simulink model "Conduction_Losses"  (R2015a)
settings: Solver=ode45  StartTime=0.0  StopTime=10.0  RelTol=1e-3
libraries: simulink x6
settings Model: Creator=Caner  LastModifiedBy=Caner

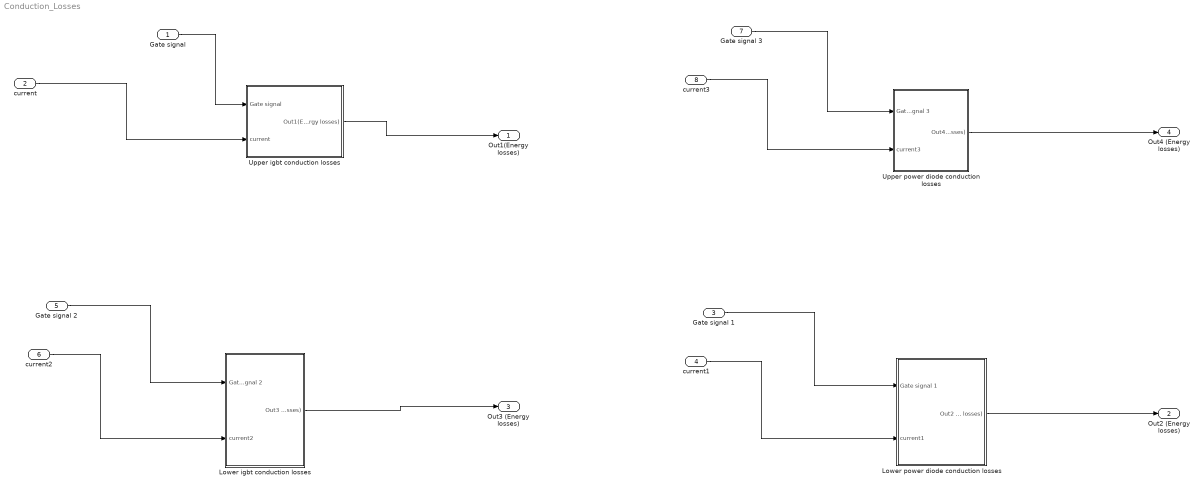
== system Conduction_Losses ==
  "Gate signal " : Inport
  current : Inport  Port=2
  Gate signal 1 : Inport  Port=3
  current1 : Inport  Port=4
  Gate signal 2 : Inport  Port=5
  current2 : Inport  Port=6
  Gate signal 3 : Inport  Port=7
  current3 : Inport  Port=8
  Lower igbt conduction losses : Subsystem
  Lower power diode conduction losses : Subsystem
  Upper igbt conduction losses : Subsystem
  Upper power diode conduction losses : Subsystem
  Out1(Energy losses) : Outport
  Out2 (Energy losses) : Outport  Port=2
  Out3 (Energy losses) : Outport  Port=3
  Out4 (Energy losses) : Outport  Port=4
  wires:
  "Gate signal "/1 -> Upper igbt conduction losses/1("Gate signal ")
  current/1 -> Upper igbt conduction losses/2(current)
  Upper igbt conduction losses/1(Out1(Energy losses)) -> Out1(Energy losses)/1
  Gate signal 2/1 -> Lower igbt conduction losses/1(Gate signal 2)
  current2/1 -> Lower igbt conduction losses/2(current2)
  Lower igbt conduction losses/1(Out3 (Energy losses)) -> Out3 (Energy losses)/1
  Gate signal 3/1 -> Upper power diode conduction losses/1(Gate signal 3)
  current3/1 -> Upper power diode conduction losses/2(current3)
  Upper power diode conduction losses/1(Out4 (Energy losses)) -> Out4 (Energy losses)/1
  Gate signal 1/1 -> Lower power diode conduction losses/1(Gate signal 1)
  current1/1 -> Lower power diode conduction losses/2(current1)
  Lower power diode conduction losses/1(Out2 (Energy losses)) -> Out2 (Energy losses)/1

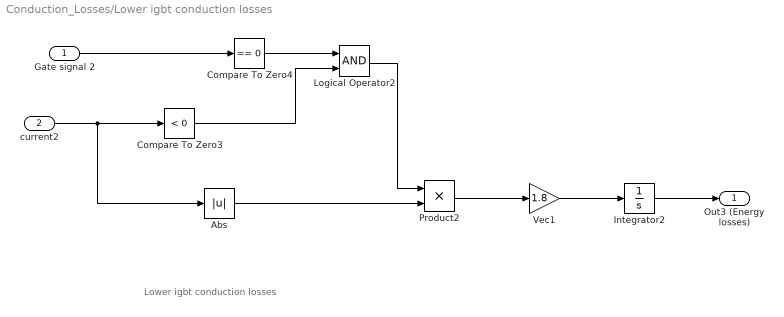
== system Conduction_Losses/Lower igbt conduction losses ==
  note: Lower igbt conduction losses
  Gate signal 2 : Inport
  current2 : Inport  Port=2
  Abs : Abs
  Compare To Zero3 : simulink/Logic and Bit Operations/Compare To Zero  relop=<  OutDataTypeStr=boolean
  Compare To Zero4 : simulink/Logic and Bit Operations/Compare To Zero  relop===  OutDataTypeStr=boolean
  Integrator2 : Integrator
  Logical Operator2 : Logic  AllPortsSameDT=off  OutDataTypeStr=boolean
  Product2 : Product
  Vec1 : Gain  Gain=1.8
  Out3 (Energy losses) : Outport
  wires:
  Gate signal 2/1 -> Compare To Zero4/1
  Compare To Zero3/1 -> Logical Operator2/2
  current2/1 -> Abs/1, Compare To Zero3/1
  Vec1/1 -> Integrator2/1
  Abs/1 -> Product2/2
  Compare To Zero4/1 -> Logical Operator2/1
  Product2/1 -> Vec1/1
  Integrator2/1 -> Out3 (Energy losses)/1
  Logical Operator2/1 -> Product2/1

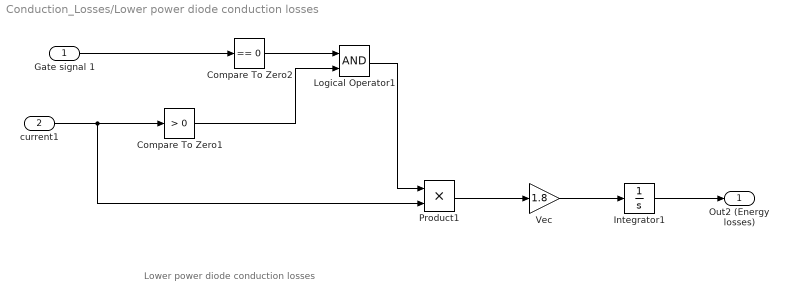
== system Conduction_Losses/Lower power diode conduction losses ==
  note: Lower power diode conduction losses
  Gate signal 1 : Inport
  current1 : Inport  Port=2
  Compare To Zero1 : simulink/Logic and Bit Operations/Compare To Zero  relop=>  OutDataTypeStr=boolean
  Compare To Zero2 : simulink/Logic and Bit Operations/Compare To Zero  relop===  OutDataTypeStr=boolean
  Integrator1 : Integrator
  Logical Operator1 : Logic  AllPortsSameDT=off  OutDataTypeStr=boolean
  Product1 : Product
  Vec : Gain  Gain=1.8
  Out2 (Energy losses) : Outport
  wires:
  Compare To Zero1/1 -> Logical Operator1/2
  Logical Operator1/1 -> Product1/1
  Gate signal 1/1 -> Compare To Zero2/1
  current1/1 -> Product1/2, Compare To Zero1/1
  Compare To Zero2/1 -> Logical Operator1/1
  Vec/1 -> Integrator1/1
  Integrator1/1 -> Out2 (Energy losses)/1
  Product1/1 -> Vec/1

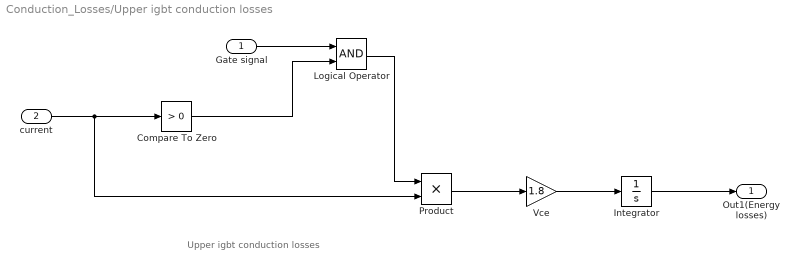
== system Conduction_Losses/Upper igbt conduction losses ==
  note: Upper igbt conduction losses
  "Gate signal " : Inport
  current : Inport  Port=2
  Compare To Zero : simulink/Logic and Bit Operations/Compare To Zero  relop=>  OutDataTypeStr=boolean
  Integrator : Integrator
  Logical Operator : Logic  AllPortsSameDT=off  OutDataTypeStr=boolean
  Product : Product
  Vce : Gain  Gain=1.8
  Out1(Energy losses) : Outport
  wires:
  Compare To Zero/1 -> Logical Operator/2
  current/1 -> Product/2, Compare To Zero/1
  Integrator/1 -> Out1(Energy losses)/1
  "Gate signal "/1 -> Logical Operator/1
  Product/1 -> Vce/1
  Vce/1 -> Integrator/1
  Logical Operator/1 -> Product/1

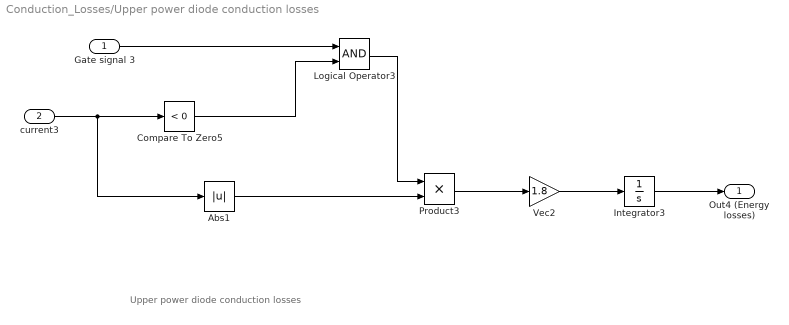
== system Conduction_Losses/Upper power diode conduction losses ==
  note: Upper power diode conduction losses
  Gate signal 3 : Inport
  current3 : Inport  Port=2
  Abs1 : Abs
  Compare To Zero5 : simulink/Logic and Bit Operations/Compare To Zero  relop=<  OutDataTypeStr=boolean
  Integrator3 : Integrator
  Logical Operator3 : Logic  AllPortsSameDT=off  OutDataTypeStr=boolean
  Product3 : Product
  Vec2 : Gain  Gain=1.8
  Out4 (Energy losses) : Outport
  wires:
  Product3/1 -> Vec2/1
  current3/1 -> Abs1/1, Compare To Zero5/1
  Abs1/1 -> Product3/2
  Compare To Zero5/1 -> Logical Operator3/2
  Gate signal 3/1 -> Logical Operator3/1
  Vec2/1 -> Integrator3/1
  Integrator3/1 -> Out4 (Energy losses)/1
  Logical Operator3/1 -> Product3/1
